simulink model "simCreateKinematicsNL"  (Simulink 7.4)
settings: Solver=ode3  StartTime=0.0  StopTime=t(end)  FixedStep=0.0001  RelTol=1e-3
undefined symbols (not defined in the file or in its folder): X0
settings Model: Creator=Jon  LastModifiedBy=Jon

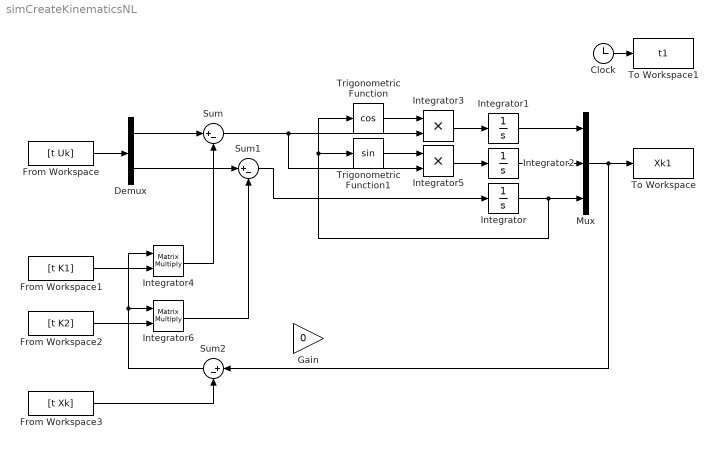
== system simCreateKinematicsNL ==
  Clock : Clock
      settings: Decimation=10
  Demux : Demux  Outputs=2
  From Workspace : FromWorkspace  VariableName=[t Uk]  SampleTime=0
  From Workspace1 : FromWorkspace  VariableName=[t K1]  SampleTime=0
  From Workspace2 : FromWorkspace  VariableName=[t K2]  SampleTime=0
  From Workspace3 : FromWorkspace  VariableName=[t Xk]  SampleTime=0
  Gain : Gain  Gain=0  ParameterDataType=fixdt(1, 16)  ParameterScaling=2^0  OutDataType=fixdt(1, 16)  OutScaling=2^0
  Integrator : Integrator  InitialCondition=X0(3)
  Integrator1 : Integrator  InitialCondition=X0(1)
  Integrator2 : Integrator  InitialCondition=X0(2)
  Integrator3 : Product  OutDataType=fixdt(1, 16)  OutScaling=2^0  RndMeth=Zero
  Integrator4 : Product  Multiplication=Matrix(*)  OutDataType=fixdt(1, 16)  OutScaling=2^0  RndMeth=Zero
  Integrator5 : Product  OutDataType=fixdt(1, 16)  OutScaling=2^0  RndMeth=Zero
  Integrator6 : Product  Multiplication=Matrix(*)  OutDataType=fixdt(1, 16)  OutScaling=2^0  RndMeth=Zero
  Mux : Mux  Inputs=3
  Sum : Sum  Inputs=|+-  OutDataType=fixdt(1, 16)  OutScaling=2^0
  Sum1 : Sum  Inputs=|+-  OutDataType=fixdt(1, 16)  OutScaling=2^0
  Sum2 : Sum  Inputs=|+-  OutDataType=fixdt(1, 16)  OutScaling=2^0
  To Workspace : ToWorkspace  VariableName=Xk1  SampleTime=-1  SaveFormat=Array
  To Workspace1 : ToWorkspace  VariableName=t1  SampleTime=-1  SaveFormat=Array
  Trigonometric Function : Trigonometry  Operator=cos
  Trigonometric Function1 : Trigonometry
  wires:
  From Workspace/1 -> Demux/1
  Trigonometric Function/1 -> Integrator3/1
  Sum/1 -> Integrator3/2, Integrator5/2
  Trigonometric Function1/1 -> Integrator5/1
  Integrator3/1 -> Integrator1/1
  Integrator5/1 -> Integrator2/1
  Integrator/1 -> Trigonometric Function1/1, Trigonometric Function/1, Mux/3
  Sum1/1 -> Integrator/1
  Integrator1/1 -> Mux/1
  Integrator2/1 -> Mux/2
  Mux/1 -> To Workspace/1, Sum2/1
  Clock/1 -> To Workspace1/1
  From Workspace1/1 -> Integrator4/2
  From Workspace2/1 -> Integrator6/2
  Demux/1 -> Sum/1
  Demux/2 -> Sum1/1
  Integrator4/1 -> Sum/2
  Integrator6/1 -> Sum1/2
  From Workspace3/1 -> Sum2/2
  Sum2/1 -> Integrator6/1, Integrator4/1
